simulink model "ident1"  (Simulink 4.00)
settings: Solver=ode45  StartTime=0.0  StopTime=30  MaxStep=0.1  RelTol=1e-3
values from neighbouring files (symbols this model uses):
  k = 0.998681225655    [ident21.mat]    (also in ncd_kalm_1.mat = [20.04 41.6748 91.25676 100.22352 54.94452 22.0392]; ncd_kalm_2.mat = [20.04 41.6748 91.25676 100.22352 54.94452 22.0392]; ncd_pol1.m = place(A, B, p); ncd_pol_1.mat = [20.04 41.6748 91.25676 100.22352 54.94452 22.0392])
  tau = 1.00031317223    [ident21.mat]
  zetha = 0.0500614532492    [ident21.mat]
settings Model: LastModifiedBy=Administrator  BlockReductionOpt=off

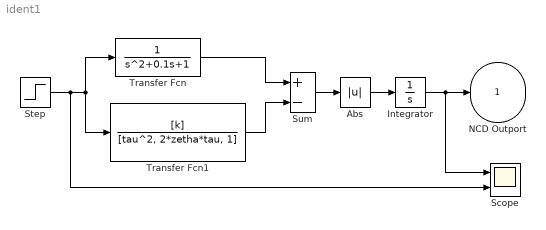
== system ident1 ==
  Abs : Abs  SaturateOnIntegerOverflow=on
  Integrator : Integrator  ExternalReset=none  InitialConditionSource=internal  InitialCondition=0  LimitOutput=off  UpperSaturationLimit=inf  LowerSaturationLimit=-inf  ShowSaturationPort=off  ShowStatePort=off  AbsoluteTolerance=auto
  Scope : Scope  NumInputPorts=2
      settings: TimeRange=auto  YMin=-1~1.16495  YMax=1~1.16495  SaveToWorkspace=off  SaveName=ScopeData  LimitDataPoints=on  MaxDataPoints=5000
  Step : Step  Time=0  Before=0  After=1  SampleTime=0
  Sum : Sum  Inputs=+-  SaturateOnIntegerOverflow=on
  Transfer Fcn : TransferFcn  Numerator=[1]  Denominator=[1 0.1 1]  Realization=auto  AbsoluteTolerance=auto
  Transfer Fcn1 : TransferFcn  Numerator=[k]  Denominator=[tau^2, 2*zetha*tau, 1]  Realization=auto  AbsoluteTolerance=auto
  NCD Outport : Outport  Port=1  InitialOutput=0
      settings: OpenFcn=optblock
      mask Type: NCD Outport
      mask Display:
      | plot([0:10],[-.5 1.5 .6 1.3 .8 1.1 .95 1.02 .99 1 1]);
      | disp('\n\n NCD\n OutPort 1');
  wires:
  Step/1 -> Transfer Fcn1/1, Transfer Fcn/1, Scope/2
  Transfer Fcn/1 -> Sum/1
  Transfer Fcn1/1 -> Sum/2
  Sum/1 -> Abs/1
  Abs/1 -> Integrator/1
  Integrator/1 -> NCD Outport/1, Scope/1
